simulink model "ejercicio14_11"  (R2016a)
settings: Solver=VariableStepAuto  StartTime=0.0  StopTime=0.01  RelTol=1e-3
undefined symbols (not defined in the file or in its folder): C, L, R
settings Model: Creator=Estudiantes  LastModifiedBy=Estudiantes

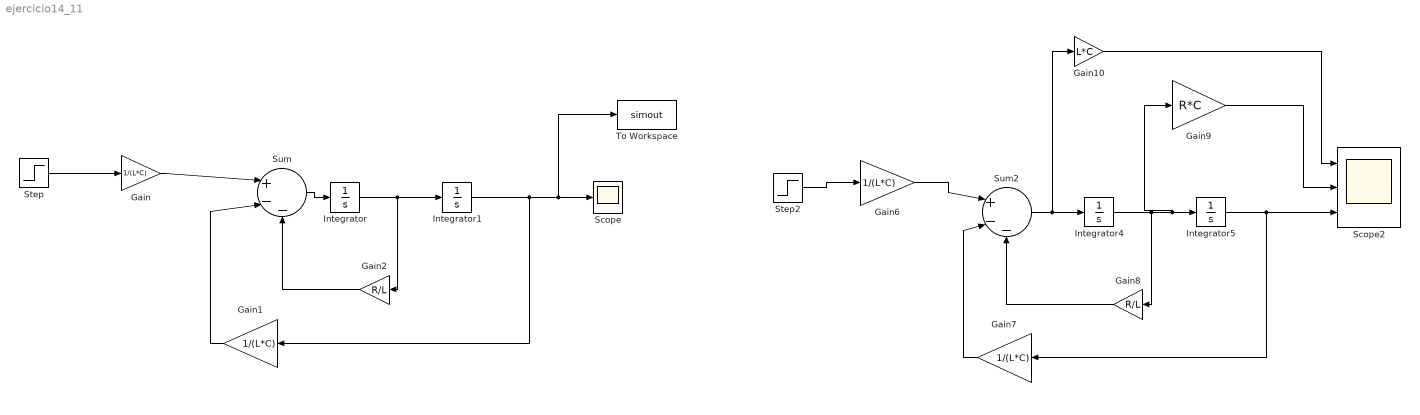
== system ejercicio14_11 ==
  Gain{,1,6..7} (4 alike) : Gain  Gain=1/(L*C)
  Gain10 : Gain  Gain=L*C
  Gain2 : Gain  Gain=R/L
  Gain8 : Gain  Gain=R/L
  Gain9 : Gain  Gain=R*C
  Integrator{,1,4..5} (4 alike) : Integrator
  Scope : Scope
  Scope2 : Scope  NumInputPorts=3
  Step : Step  Time=0  SampleTime=0
  Step2 : Step  Time=0  SampleTime=0
  Sum : Sum  Inputs=|+--
  Sum2 : Sum  Inputs=|+--
  To Workspace : ToWorkspace  VariableName=simout  SaveFormat=Timeseries  SampleTime=-1
  wires:
  Gain/1 -> Sum/1
  Gain1/1 -> Sum/2
  Gain2/1 -> Sum/3
  Sum/1 -> Integrator/1
  Integrator1/1 -> To Workspace/1, Scope/1, Gain1/1
  Step/1 -> Gain/1
  Integrator/1 -> Gain2/1, Integrator1/1
  Gain6/1 -> Sum2/1
  Gain7/1 -> Sum2/2
  Gain8/1 -> Sum2/3
  Sum2/1 -> Gain10/1, Integrator4/1
  Integrator5/1 -> Scope2/3, Gain7/1
  Step2/1 -> Gain6/1
  Integrator4/1 -> Gain8/1, Gain9/1, Integrator5/1
  Gain10/1 -> Scope2/1
  Gain9/1 -> Scope2/2
